simulink model "NOx_SCR_MIL_SIl_Model"  (R2019a)
settings: Solver=FixedStepDiscrete  StartTime=0.0  StopTime=500  FixedStep=0.1  RelTol=1e-3
undefined symbols (not defined in the file or in its folder): Actual_Injector_on, Flow_rate_min, Injector_off, injector_On_counter, Req_Downstrem_nox, Req_ON, Req_SCR_Bed_temp, Required_injector_On, Required_pressure, sigbuilder_block
settings Model: Creator=Kore  LastModifiedBy=Kore
settings ConfigComp: CovEnable=on  RecordCoverage=on  CovMetricSettings=dcmwe  CovModelRefEnable=on

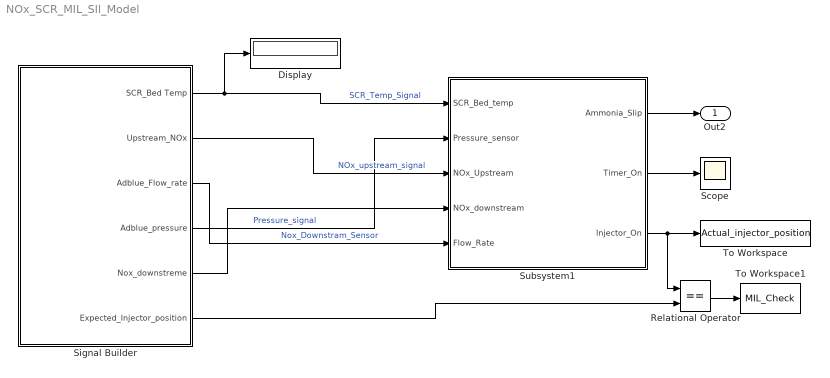
== system NOx_SCR_MIL_SIl_Model ==
  Display : Display
  Relational Operator : RelationalOperator  Operator===  OutDataTypeStr=boolean  RndMeth=Simplest
  Scope : Scope
  Signal Builder : Subsystem  Tag=STV Subsys  LoadFcn=sigbuilder_block('load');  StartFcn=sigbuilder_block('start');  StopFcn=sigbuilder_block('stop');  ClipboardFcn=sigbuilder_block('clipboard');  mask(Sigbuilder block){tuvar=[0:10]}
      mask help: Simulink:masks:SigbuilderBlock_MD
      mask init:
      | if ~strcmp(get_param(bdroot(gcbh),'SimulationStatus'),'stopped') tuvar = sigbuilder_block('maskInit'); end
      settings: CopyFcn=sigbuilder_block('copy');  DeleteFcn=sigbuilder_block('delete');  ModelCloseFcn=sigbuilder_block('modelClose');  PreSaveFcn=sigbuilder_block('preSave');  PauseFcn=sigbuilder_block('pause');  ContinueFcn=sigbuilder_block('continue');  NameChangeFcn=sigbuilder_block('namechange');  OpenFcn=sigbuilder_block('open',[437.6 153 550.4 359.25 ]);  CloseFcn=sigbuilder_block('close');
      mask Display: plot(0, 0, 100, 100,[2, 2, 32, 32, 2], [68, 8, 8, 68, 68],[32, 2], [38, 38], [32, 19, 2],[53, 60, 44], [32, 17, 17, 2],[16, 16, 31, 31]);txt = getActiveGroup(gcbh);text(2, 100, txt,'verticalAlignment', 'top');
  Subsystem1 : Subsystem
  To Workspace : ToWorkspace  VariableName=Actual_injector_position  SaveFormat=Timeseries  SampleTime=-1
  To Workspace1 : ToWorkspace  VariableName=MIL_Check  SaveFormat=Timeseries  SampleTime=-1
  Out2 : Outport
  wires:
  Subsystem1/3(Injector_On) -> Relational Operator/1, To Workspace/1
  Signal Builder/1(SCR_Bed Temp) -> Display/1, Subsystem1/1(SCR_Bed_temp)  "SCR_Temp_Signal"
  Subsystem1/1(Ammonia_Slip) -> Out2/1
  Signal Builder/2(Upstream_NOx) -> Subsystem1/3(NOx_Upstream)  "NOx_upstream_signal"
  Signal Builder/4(Adblue_pressure) -> Subsystem1/2(Pressure_sensor)  "Pressure_signal"
  Subsystem1/2(Timer_On) -> Scope/1
  Relational Operator/1 -> To Workspace1/1
  Signal Builder/6(Expected_Injector_position) -> Relational Operator/2
  Signal Builder/5(Nox_downstreme) -> Subsystem1/4(NOx_downstream)
  Signal Builder/3(Adblue_Flow_rate) -> Subsystem1/5(Flow_Rate)  "Nox_Downstram_Sensor"

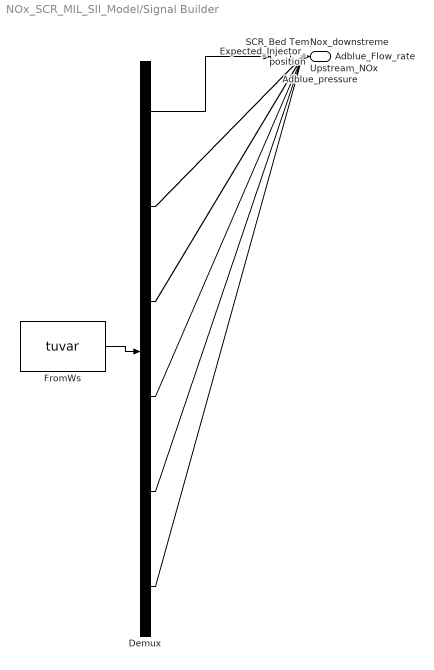
== system NOx_SCR_MIL_SIl_Model/Signal Builder ==
  Demux : Demux  Tag=STV Demux  Outputs=6
  FromWs : FromWorkspace  Tag=STV FromWs  VariableName=tuvar  SampleTime=0
      SigBuilderData=|
      | common.afterFinalStr = 'Extrapolate'
      | common.sampleTime = 0
      | dataSet.timeRange = [0 35.9]
      | dataSet.name = 'Sheet1'
      | sbobj.Name = 'Signal Builder'
      | sbobj.Groups.Name = 'Sheet1'
      | sbobj.Groups.Signals(1).Name = 'SCR_Bed Temp'
      | sbobj.Groups.Signals(1).XData = [0 0.1 0.2 0.3 0.4 0.5 0.6 0.7 0.8 0.9 1 1.1 1.2 1.3 1.4 1.5 1.6 1.7 1.8 1.9 2 2.1 2.2 2.3 2.4 2.5 2.6 2.7 2.8 2.9 3 3.1 3.2 3.3 3.4 3.5 3.6 3.7 3.8 3.9 4 4.1 4.2 4.3 4.4 4.5 4.6 4.7 4.8 4.9 5 5.1 5.2 5.3 5.4 5.5 5.6 5.7 5.8 5.9 6 6.1 6.2 6.3 6.4 6.5 6.6 6.7 6.8 6.9 7 7.1 7.2 7.3 7.4 7.5 7.6 7.7 7.8 7.9 8 8.1 8.2 8.3 8.4 8.5 8.6 8.7 8.8 8.9 9 9.1 9.2 9.3 9.4 9.5 9.6 9.7 9.8 9.9 10 10.1 10.2 10.3 10.4 10.5 10.6 10.7 10.8 10.9 11 11.1 11.2 11.3 11.4 11.5 11.6 11.7 11.8 11.9 12 12.1 12.2 12.3 12.4 12.5 12.6 12.7 12.8 12.9 13 13.1 13.2 13.3 13.4 13.5 13.6 13.7 13.8 13.9 14 14.1 14.2 14.3 14.4 14.5 14.6 14.7 14.8 14.9 15 15.1 15.2 15.3 15.4 15.5 15.6 15.7 15.8 15.9 16 16.1 16.2 16.3 16.4 16.5 16.6 16.7 16.8 16.9 17 17.1 17.2 17.3 17.4 17.5 17.6 17.7 17.8 17.9 18 18.1 18.2 18.3 18.4 18.5 18.6 18.7 18.8 18.9 19 19.1 19.2 19.3 19.4 19.5 19.6 19.7 19.8 19.9 20 20.1 20.2 20.3 20.4 20.5 20.6 20.7 20.8 20.9 21 21.1 21.2 21.3 21.4 21.5 21.6 21.7 21.8 21.9 22 22.1 22.2 22.3 22.4 22.5 22.6 22.7 22.8 22.9 23 23.1 23.2 23.3 23.4 23.5 23.6 23.7 23.8 23.9 24 24.1 24.2 24.3 24.4 24.5 24.6 24.7 24.8 24.9 25 25.1 25.2 25.3 25.4 25.5 25.6 25.7 25.8 25.9 26 26.1 26.2 26.3 26.4 26.5 26.6 26.7 26.8 26.9 27 27.1 27.2 27.3 27.4 27.5 27.6 27.7 27.8 27.9 28 28.1 28.2 28.3 28.4 28.5 28.6 28.7 28.8 28.9 29 29.1 29.2 29.3 29.4 29.5 29.6 29.7 29.8 29.9 30 30.1 30.2 30.3 30.4 30.5 30.6 30.7 30.8 30.9 31 31.1 31.2 31.3 31.4 31.5 31.6 31.7 31.8 31.9 32 32.1 32.2 32.3 32.4 32.5 32.6 32.7 32.8 32.9 33 33.1 33.2 33.3 33.4 33.5 33.6 33.7 33.8 33.9 34 34.1 34.2 34.3 34.4 34.5 34.6 34.7 34.8 34.9 35 35.1 35.2 35.3 35.4 35.5 35.6 35.7 35.8 35.9]
      | sbobj.Groups.Signals(1).YData = [1 10 20 30 40 50 60 70 80 90 100 110 120 130 140 150 160 170 180 190 200 210 220 230 240 250 260 270 280 290 300 310 320 330 340 350 360 370 380 390 400 410 420 430 440 450 460 470 480 490 500 510 520 530 540 550 560 570 580 590 600 610 620 630 640 650 660 670 10 20 30 40 50 60 70 80 90 100 110 120 130 140 150 160 170 180 190 200 210 220 230 240 250 260 270 280 290 300 310 320 330 340 350 360 370 380 390 400 410 420 430 440 450 460 470 480 490 500 510 520 530 540 550 560 570 580 590 600 610 620 630 640 650 660 670 10 20 30 40 50 60 70 80 90 100 110 120 130 140 150 160 170 180 190 200 210 220 230 240 250 260 270 280 290 300 310 320 330 340 350 360 370 380 390 400 410 420 430 440 450 460 470 480 490 500 510 520 530 540 550 560 570 580 590 600 610 620 630 640 650 660 670 10 20 30 40 50 60 70 80 90 100 110 120 130 140 150 160 170 180 190 200 210 220 230 240 250 260 270 280 290 300 310 320 330 340 350 360 370 380 390 400 410 420 430 440 450 460 470 480 490 500 510 520 530 540 550 560 570 580 590 600 610 620 630 640 650 660 670 200 205 210 215 220 225 230 235 240 245 250 255 260 265 270 275 280 285 290 295 300 305 310 315 320 325 330 335 340 345 350 355 360 365 370 375 380 385 390 395 400 405 410 415 420 425 430 435 440 445 450 455 460 465 470 475 480 485 490 495 500 505 510 515 520 525 530 535 540 545 550 555 560 565 570 575 580 585 590 595 600 605 610 615 620 625 630 635 640 645 650]
      | sbobj.Groups.Signals(2).Name = 'Upstream_NOx'
      | sbobj.Groups.Signals(2).XData = [0 0.1 0.2 0.3 0.4 0.5 0.6 0.7 0.8 0.9 1 1.1 1.2 1.3 1.4 1.5 1.6 1.7 1.8 1.9 2 2.1 2.2 2.3 2.4 2.5 2.6 2.7 2.8 2.9 3 3.1 3.2 3.3 3.4 3.5 3.6 3.7 3.8 3.9 4 4.1 4.2 4.3 4.4 4.5 4.6 4.7 4.8 4.9 5 5.1 5.2 5.3 5.4 5.5 5.6 5.7 5.8 5.9 6 6.1 6.2 6.3 6.4 6.5 6.6 6.7 6.8 6.9 7 7.1 7.2 7.3 7.4 7.5 7.6 7.7 7.8 7.9 8 8.1 8.2 8.3 8.4 8.5 8.6 8.7 8.8 8.9 9 9.1 9.2 9.3 9.4 9.5 9.6 9.7 9.8 9.9 10 10.1 10.2 10.3 10.4 10.5 10.6 10.7 10.8 10.9 11 11.1 11.2 11.3 11.4 11.5 11.6 11.7 11.8 11.9 12 12.1 12.2 12.3 12.4 12.5 12.6 12.7 12.8 12.9 13 13.1 13.2 13.3 13.4 13.5 13.6 13.7 13.8 13.9 14 14.1 14.2 14.3 14.4 14.5 14.6 14.7 14.8 14.9 15 15.1 15.2 15.3 15.4 15.5 15.6 15.7 15.8 15.9 16 16.1 16.2 16.3 16.4 16.5 16.6 16.7 16.8 16.9 17 17.1 17.2 17.3 17.4 17.5 17.6 17.7 17.8 17.9 18 18.1 18.2 18.3 18.4 18.5 18.6 18.7 18.8 18.9 19 19.1 19.2 19.3 19.4 19.5 19.6 19.7 19.8 19.9 20 20.1 20.2 20.3 20.4 20.5 20.6 20.7 20.8 20.9 21 21.1 21.2 21.3 21.4 21.5 21.6 21.7 21.8 21.9 22 22.1 22.2 22.3 22.4 22.5 22.6 22.7 22.8 22.9 23 23.1 23.2 23.3 23.4 23.5 23.6 23.7 23.8 23.9 24 24.1 24.2 24.3 24.4 24.5 24.6 24.7 24.8 24.9 25 25.1 25.2 25.3 25.4 25.5 25.6 25.7 25.8 25.9 26 26.1 26.2 26.3 26.4 26.5 26.6 26.7 26.8 26.9 27 27.1 27.2 27.3 27.4 27.5 27.6 27.7 27.8 27.9 28 28.1 28.2 28.3 28.4 28.5 28.6 28.7 28.8 28.9 29 29.1 29.2 29.3 29.4 29.5 29.6 29.7 29.8 29.9 30 30.1 30.2 30.3 30.4 30.5 30.6 30.7 30.8 30.9 31 31.1 31.2 31.3 31.4 31.5 31.6 31.7 31.8 31.9 32 32.1 32.2 32.3 32.4 32.5 32.6 32.7 32.8 32.9 33 33.1 33.2 33.3 33.4 33.5 33.6 33.7 33.8 33.9 34 34.1 34.2 34.3 34.4 34.5 34.6 34.7 34.8 34.9 35 35.1 35.2 35.3 35.4 35.5 35.6 35.7 35.8 35.9]
      | sbobj.Groups.Signals(2).YData = [10 70 77.6 80.4 86.4 99.6 108 117.6 127.2 136.8 149.3 158.3 ... (360 elements, 1x360)]
      | sbobj.Groups.Signals(3).Name = 'Adblue_Flow_rate'
      | sbobj.Groups.Signals(3).XData = [0 0.1 0.2 0.3 0.4 0.5 0.6 0.7 0.8 0.9 1 1.1 1.2 1.3 1.4 1.5 1.6 1.7 1.8 1.9 2 2.1 2.2 2.3 2.4 2.5 2.6 2.7 2.8 2.9 3 3.1 3.2 3.3 3.4 3.5 3.6 3.7 3.8 3.9 4 4.1 4.2 4.3 4.4 4.5 4.6 4.7 4.8 4.9 5 5.1 5.2 5.3 5.4 5.5 5.6 5.7 5.8 5.9 6 6.1 6.2 6.3 6.4 6.5 6.6 6.7 6.8 6.9 7 7.1 7.2 7.3 7.4 7.5 7.6 7.7 7.8 7.9 8 8.1 8.2 8.3 8.4 8.5 8.6 8.7 8.8 8.9 9 9.1 9.2 9.3 9.4 9.5 9.6 9.7 9.8 9.9 10 10.1 10.2 10.3 10.4 10.5 10.6 10.7 10.8 10.9 11 11.1 11.2 11.3 11.4 11.5 11.6 11.7 11.8 11.9 12 12.1 12.2 12.3 12.4 12.5 12.6 12.7 12.8 12.9 13 13.1 13.2 13.3 13.4 13.5 13.6 13.7 13.8 13.9 14 14.1 14.2 14.3 14.4 14.5 14.6 14.7 14.8 14.9 15 15.1 15.2 15.3 15.4 15.5 15.6 15.7 15.8 15.9 16 16.1 16.2 16.3 16.4 16.5 16.6 16.7 16.8 16.9 17 17.1 17.2 17.3 17.4 17.5 17.6 17.7 17.8 17.9 18 18.1 18.2 18.3 18.4 18.5 18.6 18.7 18.8 18.9 19 19.1 19.2 19.3 19.4 19.5 19.6 19.7 19.8 19.9 20 20.1 20.2 20.3 20.4 20.5 20.6 20.7 20.8 20.9 21 21.1 21.2 21.3 21.4 21.5 21.6 21.7 21.8 21.9 22 22.1 22.2 22.3 22.4 22.5 22.6 22.7 22.8 22.9 23 23.1 23.2 23.3 23.4 23.5 23.6 23.7 23.8 23.9 24 24.1 24.2 24.3 24.4 24.5 24.6 24.7 24.8 24.9 25 25.1 25.2 25.3 25.4 25.5 25.6 25.7 25.8 25.9 26 26.1 26.2 26.3 26.4 26.5 26.6 26.7 26.8 26.9 27 27.1 27.2 27.3 27.4 27.5 27.6 27.7 27.8 27.9 28 28.1 28.2 28.3 28.4 28.5 28.6 28.7 28.8 28.9 29 29.1 29.2 29.3 29.4 29.5 29.6 29.7 29.8 29.9 30 30.1 30.2 30.3 30.4 30.5 30.6 30.7 30.8 30.9 31 31.1 31.2 31.3 31.4 31.5 31.6 31.7 31.8 31.9 32 32.1 32.2 32.3 32.4 32.5 32.6 32.7 32.8 32.9 33 33.1 33.2 33.3 33.4 33.5 33.6 33.7 33.8 33.9 34 34.1 34.2 34.3 34.4 34.5 34.6 34.7 34.8 34.9 35 35.1 35.2 35.3 35.4 35.5 35.6 35.7 35.8 35.9]
      | sbobj.Groups.Signals(3).YData = [4 4 4 4 4 4 4 4 4 4.8 4.8 4.8 ... (360 elements, 1x360)]
      | sbobj.Groups.Signals(4).Name = 'Adblue_pressure'
      | sbobj.Groups.Signals(4).XData = [0 0.1 0.2 0.3 0.4 0.5 0.6 0.7 0.8 0.9 1 1.1 1.2 1.3 1.4 1.5 1.6 1.7 1.8 1.9 2 2.1 2.2 2.3 2.4 2.5 2.6 2.7 2.8 2.9 3 3.1 3.2 3.3 3.4 3.5 3.6 3.7 3.8 3.9 4 4.1 4.2 4.3 4.4 4.5 4.6 4.7 4.8 4.9 5 5.1 5.2 5.3 5.4 5.5 5.6 5.7 5.8 5.9 6 6.1 6.2 6.3 6.4 6.5 6.6 6.7 6.8 6.9 7 7.1 7.2 7.3 7.4 7.5 7.6 7.7 7.8 7.9 8 8.1 8.2 8.3 8.4 8.5 8.6 8.7 8.8 8.9 9 9.1 9.2 9.3 9.4 9.5 9.6 9.7 9.8 9.9 10 10.1 10.2 10.3 10.4 10.5 10.6 10.7 10.8 10.9 11 11.1 11.2 11.3 11.4 11.5 11.6 11.7 11.8 11.9 12 12.1 12.2 12.3 12.4 12.5 12.6 12.7 12.8 12.9 13 13.1 13.2 13.3 13.4 13.5 13.6 13.7 13.8 13.9 14 14.1 14.2 14.3 14.4 14.5 14.6 14.7 14.8 14.9 15 15.1 15.2 15.3 15.4 15.5 15.6 15.7 15.8 15.9 16 16.1 16.2 16.3 16.4 16.5 16.6 16.7 16.8 16.9 17 17.1 17.2 17.3 17.4 17.5 17.6 17.7 17.8 17.9 18 18.1 18.2 18.3 18.4 18.5 18.6 18.7 18.8 18.9 19 19.1 19.2 19.3 19.4 19.5 19.6 19.7 19.8 19.9 20 20.1 20.2 20.3 20.4 20.5 20.6 20.7 20.8 20.9 21 21.1 21.2 21.3 21.4 21.5 21.6 21.7 21.8 21.9 22 22.1 22.2 22.3 22.4 22.5 22.6 22.7 22.8 22.9 23 23.1 23.2 23.3 23.4 23.5 23.6 23.7 23.8 23.9 24 24.1 24.2 24.3 24.4 24.5 24.6 24.7 24.8 24.9 25 25.1 25.2 25.3 25.4 25.5 25.6 25.7 25.8 25.9 26 26.1 26.2 26.3 26.4 26.5 26.6 26.7 26.8 26.9 27 27.1 27.2 27.3 27.4 27.5 27.6 27.7 27.8 27.9 28 28.1 28.2 28.3 28.4 28.5 28.6 28.7 28.8 28.9 29 29.1 29.2 29.3 29.4 29.5 29.6 29.7 29.8 29.9 30 30.1 30.2 30.3 30.4 30.5 30.6 30.7 30.8 30.9 31 31.1 31.2 31.3 31.4 31.5 31.6 31.7 31.8 31.9 32 32.1 32.2 32.3 32.4 32.5 32.6 32.7 32.8 32.9 33 33.1 33.2 33.3 33.4 33.5 33.6 33.7 33.8 33.9 34 34.1 34.2 34.3 34.4 34.5 34.6 34.7 34.8 34.9 35 35.1 35.2 35.3 35.4 35.5 35.6 35.7 35.8 35.9]
      | sbobj.Groups.Signals(4).YData = [5.8 5.8 5.8 5.8 5.8 5.8 5.8 5.8 5.8 5.8 5.8 5.8 5.8 5.8 5.8 5.8 5.8 5.8 5.8 5.8 5.8 5.8 5.8 5.8 5.8 5.8 5.8 5.8 5.8 5.8 5.8 5.8 5.8 5.8 5.8 5.8 5.8 5.8 5.8 5.8 5.8 5.8 5.8 5.8 5.8 5.8 5.8 5.8 5.8 5.8 5.8 5.8 5.8 5.8 5.8 5.8 5.8 5.8 5.8 5.8 5.8 5.8 5.8 5.8 5.8 5.8 5.8 5.8 5.8 5.8 5.8 5.8 5.8 5.8 5.8 5.8 5.8 5.8 5.8 5.8 5.8 5.8 5.8 5.8 5.8 5.8 5.8 5.8 5.8 5.8 5.8 5.8 5.8 5.8 5.8 5.8 5.8 5.8 5.8 5.8 5.8 5.8 5.8 5.8 5.8 5.8 5.8 5.8 5.8 5.8 5.8 5.8 5.8 5.8 5.8 5.8 5.8 5.8 5.8 5.8 5.8 5.8 5.8 5.8 5.8 5.8 5.8 5.8 5.8 5.8 5.8 5.8 5.8 5.8 5.8 4.5 4.3 4.2 4.1 4.9 5 5.1 6 6.4 6.3 4.5 4.3 4.2 4.1 4.9 5 5.1 6 6.4 6.3 4.5 4.3 4.2 4.1 4.9 5 5.1 6 6.4 6.3 4.5 4.3 4.2 4.1 4.9 5 5.1 6 6.4 6.3 4.5 4.3 4.2 4.1 4.9 5 5.1 6 6.4 6.3 4.5 4.3 4.2 4.1 4.9 5 5.1 6 6.4 6.3 4.5 4.3 4.2 4.1 4.9 5 5.1 5.8 5.8 5.8 5.8 5.8 5.8 5.8 5.8 5.8 5.8 5.8 5.8 5.8 5.8 5.8 5.8 5.8 5.8 5.8 5.8 5.8 5.8 5.8 5.8 5.8 5.8 5.8 5.8 5.8 5.8 5.8 5.8 5.8 5.8 5.8 5.8 5.8 5.8 5.8 5.8 5.8 5.8 5.8 5.8 5.8 5.8 5.8 5.8 5.8 5.8 5.8 5.8 5.8 5.8 5.8 5.8 5.8 5.8 5.8 5.8 5.8 5.8 5.8 5.8 5.8 5.8 5.8 5.8 5.8 5.8 5.8 5.8 5.8 5.8 5.8 5.8 5.8 5.8 5.8 5.8 5.8 5.8 5.8 5.8 5.8 5.8 5.8 5.8 5.8 5.8 5.8 5.8 5.8 5.8 5.8 5.8 5.8 5.8 5.8 5.8 5.8 5.8 5.8 5.8 5.8 5.8 5.8 5.8 5.8 5.8 5.8 5.8 5.8 5.8 5.8 5.8 5.8 5.8 5.8 5.8 5.8 5.8 5.8 5.8 5.8 5.8 5.8 5.8 5.8 5.8 5.8 5.8 5.8 5.8 5.8 5.8 5.8 5.8 5.8 5.8 5.8 5.8 5.8 5.8 5.8 5.8 5.8 5.8 5.8 5.8 5.8 5.8 5.8 5.8 5.8 5.8 5.8 5.8]
      | sbobj.Groups.Signals(5).Name = 'Nox_downstreme'
      | sbobj.Groups.Signals(5).XData = [0 0.1 0.2 0.3 0.4 0.5 0.6 0.7 0.8 0.9 1 1.1 1.2 1.3 1.4 1.5 1.6 1.7 1.8 1.9 2 2.1 2.2 2.3 2.4 2.5 2.6 2.7 2.8 2.9 3 3.1 3.2 3.3 3.4 3.5 3.6 3.7 3.8 3.9 4 4.1 4.2 4.3 4.4 4.5 4.6 4.7 4.8 4.9 5 5.1 5.2 5.3 5.4 5.5 5.6 5.7 5.8 5.9 6 6.1 6.2 6.3 6.4 6.5 6.6 6.7 6.8 6.9 7 7.1 7.2 7.3 7.4 7.5 7.6 7.7 7.8 7.9 8 8.1 8.2 8.3 8.4 8.5 8.6 8.7 8.8 8.9 9 9.1 9.2 9.3 9.4 9.5 9.6 9.7 9.8 9.9 10 10.1 10.2 10.3 10.4 10.5 10.6 10.7 10.8 10.9 11 11.1 11.2 11.3 11.4 11.5 11.6 11.7 11.8 11.9 12 12.1 12.2 12.3 12.4 12.5 12.6 12.7 12.8 12.9 13 13.1 13.2 13.3 13.4 13.5 13.6 13.7 13.8 13.9 14 14.1 14.2 14.3 14.4 14.5 14.6 14.7 14.8 14.9 15 15.1 15.2 15.3 15.4 15.5 15.6 15.7 15.8 15.9 16 16.1 16.2 16.3 16.4 16.5 16.6 16.7 16.8 16.9 17 17.1 17.2 17.3 17.4 17.5 17.6 17.7 17.8 17.9 18 18.1 18.2 18.3 18.4 18.5 18.6 18.7 18.8 18.9 19 19.1 19.2 19.3 19.4 19.5 19.6 19.7 19.8 19.9 20 20.1 20.2 20.3 20.4 20.5 20.6 20.7 20.8 20.9 21 21.1 21.2 21.3 21.4 21.5 21.6 21.7 21.8 21.9 22 22.1 22.2 22.3 22.4 22.5 22.6 22.7 22.8 22.9 23 23.1 23.2 23.3 23.4 23.5 23.6 23.7 23.8 23.9 24 24.1 24.2 24.3 24.4 24.5 24.6 24.7 24.8 24.9 25 25.1 25.2 25.3 25.4 25.5 25.6 25.7 25.8 25.9 26 26.1 26.2 26.3 26.4 26.5 26.6 26.7 26.8 26.9 27 27.1 27.2 27.3 27.4 27.5 27.6 27.7 27.8 27.9 28 28.1 28.2 28.3 28.4 28.5 28.6 28.7 28.8 28.9 29 29.1 29.2 29.3 29.4 29.5 29.6 29.7 29.8 29.9 30 30.1 30.2 30.3 30.4 30.5 30.6 30.7 30.8 30.9 31 31.1 31.2 31.3 31.4 31.5 31.6 31.7 31.8 31.9 32 32.1 32.2 32.3 32.4 32.5 32.6 32.7 32.8 32.9 33 33.1 33.2 33.3 33.4 33.5 33.6 33.7 33.8 33.9 34 34.1 34.2 34.3 34.4 34.5 34.6 34.7 34.8 34.9 35 35.1 35.2 35.3 35.4 35.5 35.6 35.7 35.8 35.9]
      | sbobj.Groups.Signals(5).YData = [15 15 15 14 14 14 14 15 15 15 15 17 17 17 17 15 15 15 15 15 15 15 15 15 15 15 15 15 15 13 13 13 13 13 13 13 13 13 13 15 15 15 15 15 15 15 12 12 12 12 12 12 12 12 12 15 15 16 16 16 16 16 15 15 15 14 14 14 14 15 15 15 15 17 17 17 17 15 15 15 15 15 15 15 15 15 15 15 15 15 15 13 13 13 13 13 13 13 13 13 13 15 15 15 15 15 15 15 12 12 12 12 12 12 12 12 12 15 15 16 16 16 16 16 12 12 15 15 16 16 16 16 16 16 16 15 15 15 14 14 14 14 15 15 15 15 17 17 17 17 15 15 15 15 15 15 15 15 15 15 15 15 15 15 13 13 13 13 13 13 13 13 13 13 15 15 15 15 15 15 15 12 12 12 12 12 12 12 12 12 15 15 16 16 16 16 16 15 15 15 14 14 6 7 8 9 9 8 7 6 6 7 8 9 9 8 7 6 8 7 6 6 7 8 9 9 6 7 8 9 9 8 7 6 7 8 9 9 8 7 6 8 7 6 6 7 8 9 9 6 7 8 9 9 8 6 7 8 9 9 8 6 7 8 9 9 8 7 6 14 14 14 15 15 15 15 17 17 15 15 15 13 13 13 13 13 13 13 13 13 13 15 15 15 15 15 15 15 12 12 12 12 12 12 12 12 12 15 15 16 16 16 16 16 15 15 15 14 14 14 15 15 15 15 17 17 15 15 15 14 14 14 14 15 15 15 15 17 17 17 17 15 15 15 15 15 15 15 15 15 15 15 15 15 15 13 13 13 13 13]
      | sbobj.Groups.Signals(6).Name = 'Expected_Injector_position'
      | sbobj.Groups.Signals(6).XData = [0 0.1 0.2 0.3 0.4 0.5 0.6 0.7 0.8 0.9 1 1.1 1.2 1.3 1.4 1.5 1.6 1.7 1.8 1.9 2 2.1 2.2 2.3 2.4 2.5 2.6 2.7 2.8 2.9 3 3.1 3.2 3.3 3.4 3.5 3.6 3.7 3.8 3.9 4 4.1 4.2 4.3 4.4 4.5 4.6 4.7 4.8 4.9 5 5.1 5.2 5.3 5.4 5.5 5.6 5.7 5.8 5.9 6 6.1 6.2 6.3 6.4 6.5 6.6 6.7 6.8 6.9 7 7.1 7.2 7.3 7.4 7.5 7.6 7.7 7.8 7.9 8 8.1 8.2 8.3 8.4 8.5 8.6 8.7 8.8 8.9 9 9.1 9.2 9.3 9.4 9.5 9.6 9.7 9.8 9.9 10 10.1 10.2 10.3 10.4 10.5 10.6 10.7 10.8 10.9 11 11.1 11.2 11.3 11.4 11.5 11.6 11.7 11.8 11.9 12 12.1 12.2 12.3 12.4 12.5 12.6 12.7 12.8 12.9 13 13.1 13.2 13.3 13.4 13.5 13.6 13.7 13.8 13.9 14 14.1 14.2 14.3 14.4 14.5 14.6 14.7 14.8 14.9 15 15.1 15.2 15.3 15.4 15.5 15.6 15.7 15.8 15.9 16 16.1 16.2 16.3 16.4 16.5 16.6 16.7 16.8 16.9 17 17.1 17.2 17.3 17.4 17.5 17.6 17.7 17.8 17.9 18 18.1 18.2 18.3 18.4 18.5 18.6 18.7 18.8 18.9 19 19.1 19.2 19.3 19.4 19.5 19.6 19.7 19.8 19.9 20 20.1 20.2 20.3 20.4 20.5 20.6 20.7 20.8 20.9 21 21.1 21.2 21.3 21.4 21.5 21.6 21.7 21.8 21.9 22 22.1 22.2 22.3 22.4 22.5 22.6 22.7 22.8 22.9 23 23.1 23.2 23.3 23.4 23.5 23.6 23.7 23.8 23.9 24 24.1 24.2 24.3 24.4 24.5 24.6 24.7 24.8 24.9 25 25.1 25.2 25.3 25.4 25.5 25.6 25.7 25.8 25.9 26 26.1 26.2 26.3 26.4 26.5 26.6 26.7 26.8 26.9 27 27.1 27.2 27.3 27.4 27.5 27.6 27.7 27.8 27.9 28 28.1 28.2 28.3 28.4 28.5 28.6 28.7 28.8 28.9 29 29.1 29.2 29.3 29.4 29.5 29.6 29.7 29.8 29.9 30 30.1 30.2 30.3 30.4 30.5 30.6 30.7 30.8 30.9 31 31.1 31.2 31.3 31.4 31.5 31.6 31.7 31.8 31.9 32 32.1 32.2 32.3 32.4 32.5 32.6 32.7 32.8 32.9 33 33.1 33.2 33.3 33.4 33.5 33.6 33.7 33.8 33.9 34 34.1 34.2 34.3 34.4 34.5 34.6 34.7 34.8 34.9 35 35.1 35.2 35.3 35.4 35.5 35.6 35.7 35.8 35.9]
      | sbobj.Groups.Signals(6).YData = [0 0 0 0 0 0 0 0 0 0 0 0 0 0 0 0 0 0 0 0 1 1 1 1 1 1 1 1 1 1 1 1 1 1 1 1 1 1 1 1 1 1 1 1 1 1 1 1 1 1 1 1 1 1 1 1 1 1 1 1 1 1 1 1 1 1 1 1 0 0 0 0 0 0 0 0 0 0 0 0 0 0 0 0 0 0 0 0 0 0 0 0 0 0 0 0 0 0 0 0 0 0 0 0 0 0 0 0 0 0 0 0 0 0 0 0 0 0 0 0 0 0 0 0 0 0 0 0 0 0 0 0 0 0 0 0 0 0 0 0 0 0 0 0 0 0 0 0 0 0 0 0 0 0 0 0 0 0 0 0 0 0 0 0 0 0 0 0 0 0 0 0 0 0 0 0 0 0 0 0 0 0 0 0 0 0 0 0 0 0 0 0 0 0 0 0 0 0 0 0 0 0 0 0 0 0 0 0 0 0 0 0 0 0 0 0 0 0 0 0 0 0 0 0 0 0 0 0 0 0 0 0 0 0 0 0 0 0 0 0 0 0 0 0 0 0 0 0 0 0 0 0 0 0 0 0 0 0 0 0 0 0 0 0 0 0 0 0 0 1 1 1 1 1 1 1 1 1 1 1 1 1 1 1 1 1 1 1 1 1 1 1 1 1 1 1 1 1 1 1 1 1 1 1 1 1 1 1 1 1 1 1 1 1 1 1 1 1 1 1 1 1 1 1 1 1 1 1 1 1 1 1 1 1 1 1 1 1 1 1 1 1 1 1 1 1 1 1 1 1 1 1 1 1 1 1 1 1 1 1]
      | sbobj.Groups.TimeRange = [0 35.9]
  SCR_Bed Temp : Outport  Tag=STV Outport
  Upstream_NOx : Outport  Tag=STV Outport  Port=2
  Adblue_Flow_rate : Outport  Tag=STV Outport  Port=3
  Adblue_pressure : Outport  Tag=STV Outport  Port=4
  Nox_downstreme : Outport  Tag=STV Outport  Port=5
  Expected_Injector_position : Outport  Tag=STV Outport  Port=6
  wires:
  Demux/1 -> SCR_Bed Temp/1
  FromWs/1 -> Demux/1
  Demux/2 -> Upstream_NOx/1
  Demux/3 -> Adblue_Flow_rate/1
  Demux/4 -> Adblue_pressure/1
  Demux/5 -> Nox_downstreme/1
  Demux/6 -> Expected_Injector_position/1

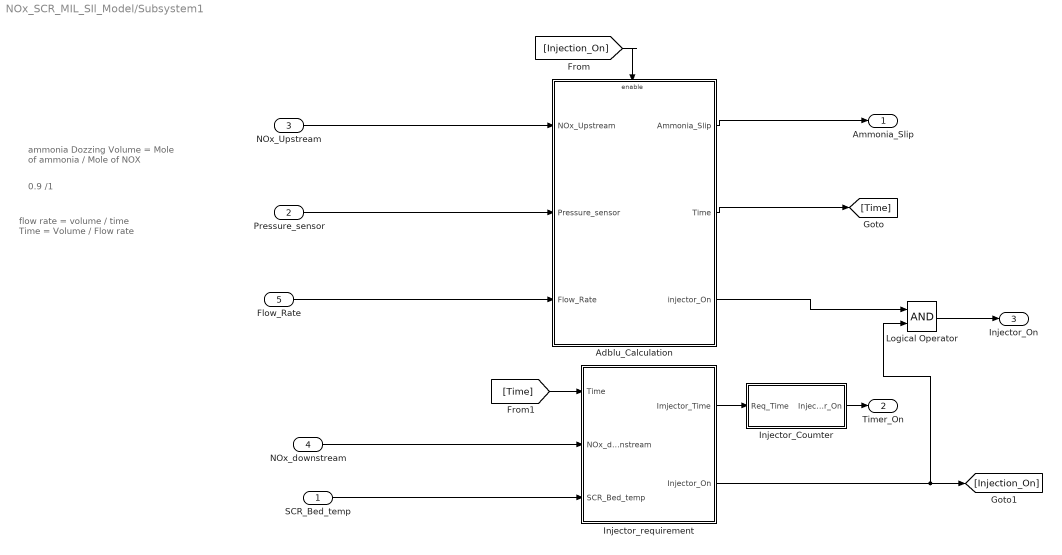
== system NOx_SCR_MIL_SIl_Model/Subsystem1 ==
  note: 0.9 /1
  note: ammonia Dozzing Volume =
      |  Mole of ammonia / Mole of NOX
  note: flow rate = volume / time
      |
      | Time = Volume / Flow rate
  SCR_Bed_temp : Inport
  Pressure_sensor : Inport  Port=2
  NOx_Upstream : Inport  Port=3
  NOx_downstream : Inport  Port=4
  Flow_Rate : Inport  Port=5
  Adblu_Calculation : Subsystem
  Injector_Coumter : Subsystem
  Injector_requirement : Subsystem
  Logical Operator : Logic  AllPortsSameDT=off  OutDataTypeStr=boolean
  Ammonia_Slip : Outport
  Timer_On : Outport  Port=2
  Injector_On : Outport  Port=3
  wires:
  NOx_Upstream/1 -> Adblu_Calculation/1(NOx_Upstream)
  Pressure_sensor/1 -> Adblu_Calculation/2(Pressure_sensor)
  Adblu_Calculation/1(Ammonia_Slip) -> Ammonia_Slip/1
  NOx_downstream/1 -> Injector_requirement/2(NOx_downstream)
  [Injection_On] -> Adblu_Calculation/Enable
  Injector_Coumter/1(Injector_On) -> Timer_On/1
  SCR_Bed_temp/1 -> Injector_requirement/3(SCR_Bed_temp)
  Injector_requirement/1(Imjector_Time) -> Injector_Coumter/1(Req_Time)
  Adblu_Calculation/2(Time) -> [Time]
  [Time] -> Injector_requirement/1(Time)
  Injector_requirement/2(Injector_On) -> Logical Operator/2, [Injection_On]
  Flow_Rate/1 -> Adblu_Calculation/3(Flow_Rate)
  Adblu_Calculation/3(injector_On) -> Logical Operator/1
  Logical Operator/1 -> Injector_On/1

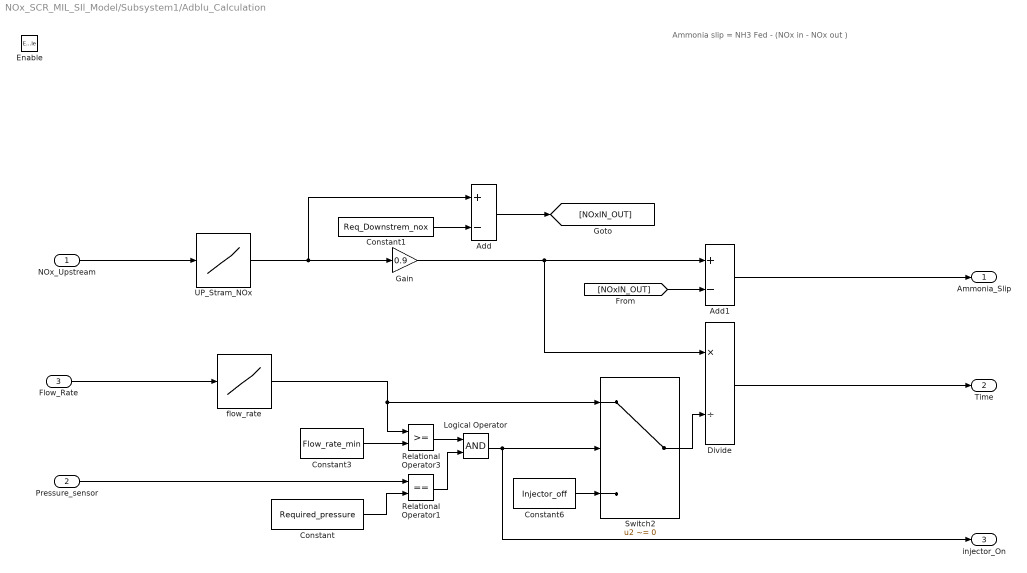
== system NOx_SCR_MIL_SIl_Model/Subsystem1/Adblu_Calculation ==
  note: Ammonia slip = NH3 Fed - (NOx in - NOx out )
  NOx_Upstream : Inport
  Pressure_sensor : Inport  Port=2
  Flow_Rate : Inport  Port=3
  Enable : EnablePort  StatesWhenEnabling=reset
  Add : Sum  Inputs=+-
  Add1 : Sum  Inputs=+-
  Constant : Constant  Value=Required_pressure
  Constant1 : Constant  Value=Req_Downstrem_nox
  Constant3 : Constant  Value=Flow_rate_min
  Constant6 : Constant  Value=Injector_off
  Divide : Product  Inputs=*/  OutDataTypeStr=double  RndMeth=Round
  Gain : Gain  Gain=0.9
  Logical Operator : Logic  AllPortsSameDT=off  OutDataTypeStr=boolean
  Relational Operator1 : RelationalOperator  Operator===  OutDataTypeStr=boolean  RndMeth=Simplest
  Relational Operator3 : RelationalOperator  OutDataTypeStr=boolean  RndMeth=Simplest
  Switch2 : Switch  Criteria=u2 ~= 0
  UP_Stram_NOx : Lookup_n-D  NumberOfTableDimensions=1  BreakpointsForDimension1=[1:5:650]  BreakpointsForDimension2=[1:1:500]  BreakpointsForDimension1DataTypeStr=double  Table=[1:5:650]  TableDataTypeStr=double  IntermediateResultsDataTypeStr=double  InternalRulePriority=Speed  OutDataTypeStr=double  RndMeth=Simplest  FractionDataTypeStr=double  InputSameDT=on
  flow_rate : Lookup_n-D  NumberOfTableDimensions=1  BreakpointsForDimension1=|  BreakpointsForDimension2=[1:1:500]  BreakpointsForDimension1DataTypeStr=double  Table=|  TableDataTypeStr=double  IntermediateResultsDataTypeStr=double  InternalRulePriority=Speed  OutDataTypeStr=double  RndMeth=Simplest  FractionDataTypeStr=double  InputSameDT=on
      BreakpointsForDimension1=|
      | [10
      | 70
      | 77.6
      | 80.4
      | 86.4
      | 99.6
      | 108
      | 117.6
      | 127.2
      | 136.8
      | 149.3
      | 158.3
      | 163.3
      | 168.3
      | 175.3
      | 181.5
      | 187.7
      | 193.9
      | 200.1
      | 206.3
      | 212.85
      | 223.5
      | 233.15
      | 242.8
      | 255.45
      | 264.9
      | 275.35
      | 285.8
      | 296.25
      | 306.7
      | 317.15
      | 327.6
      | 338.05
      | 348.5
      | 358.95
      | 369.4
      | 379.85
      | 390.3
      | 400.75
      | 411.2
      | 421.65
      | 432.1
      | 442.55
      | 453
      | 463.45
      | 473.9
      | 484.35
      | 494.8
      | 505.25
      | 515.7
      | 526.15
      | 536.6
      | 547.05
      | 557.5
      | 567.95
      | 578.4
      | 588.85
      | 599.3
      | 609.75
      | 620.2
      | 630.65
      | 641.1
      | 651.55
      | 662
      | 672.45
      | 682.9
      | 693.35
      | 703.8
      | ]
      Table=|
      | [3
      | 3
      | 3
      | 3
      | 3
      | 4
      | 4
      | 4
      | 4
      | 4.8
      | 4.8
      | 4.8
      | 4.8
      | 4.8
      | 4.8
      | 4.8
      | 4.8
      | 4.8
      | 4.8
      | 4.8
      | 4.8
      | 5.8
      | 6.4
      | 7.3
      | 8.1
      | 8.9
      | 9.7
      | 10.5
      | 11.3
      | 12.1
      | 12.9
      | 13.7
      | 14.5
      | 15.3
      | 16.1
      | 16.9
      | 17.7
      | 18.5
      | 19.3
      | 20.1
      | 20.9
      | 21.7
      | 22.5
      | 23.3
      | 24.1
      | 24.9
      | 25.7
      | 26.5
      | 27.3
      | 27.3
      | 27.3
      | 28.1
      | 28.1
      | 28.1
      | 28.1
      | 28.9
      | 28.9
      | 28.9
      | 28.9
      | 28.9
      | 28.9
      | 29.7
      | 29.7
      | 29.7
      | 29.7
      | 30.0
      | 30.0
      | 30.0]
  Ammonia_Slip : Outport
  Time : Outport  Port=2
  injector_On : Outport  Port=3
  wires:
  Pressure_sensor/1 -> Relational Operator1/1
  Add/1 -> [NOxIN_OUT]
  Constant1/1 -> Add/2
  Relational Operator1/1 -> Logical Operator/2
  Constant/1 -> Relational Operator1/2
  UP_Stram_NOx/1 -> Gain/1, Add/1
  Constant3/1 -> Relational Operator3/2
  Relational Operator3/1 -> Logical Operator/1
  Constant6/1 -> Switch2/3
  Switch2/1 -> Divide/2
  Logical Operator/1 -> injector_On/1, Switch2/2
  [NOxIN_OUT] -> Add1/2
  flow_rate/1 -> Relational Operator3/1, Switch2/1
  NOx_Upstream/1 -> UP_Stram_NOx/1
  Add1/1 -> Ammonia_Slip/1
  Gain/1 -> Divide/1, Add1/1
  Divide/1 -> Time/1
  Flow_Rate/1 -> flow_rate/1

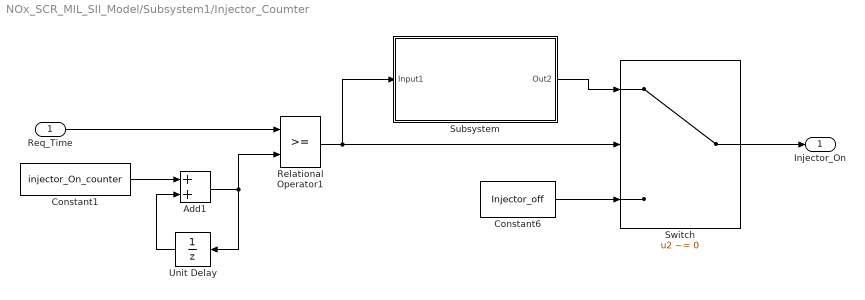
== system NOx_SCR_MIL_SIl_Model/Subsystem1/Injector_Coumter ==
  Req_Time : Inport
  Add1 : Sum
  Constant1 : Constant  Value=injector_On_counter
  Constant6 : Constant  Value=Injector_off
  Relational Operator1 : RelationalOperator  OutDataTypeStr=boolean  RndMeth=Simplest
  Subsystem : Subsystem
  Switch : Switch  Criteria=u2 ~= 0
  Unit Delay : UnitDelay  SampleTime=-1  HasFrameUpgradeWarning=on
  Injector_On : Outport
  wires:
  Constant6/1 -> Switch/3
  Unit Delay/1 -> Add1/2
  Constant1/1 -> Add1/1
  Add1/1 -> Unit Delay/1, Relational Operator1/2
  Subsystem/1(Out2) -> Switch/1
  Req_Time/1 -> Relational Operator1/1
  Switch/1 -> Injector_On/1
  Relational Operator1/1 -> Subsystem/1(Input1), Switch/2

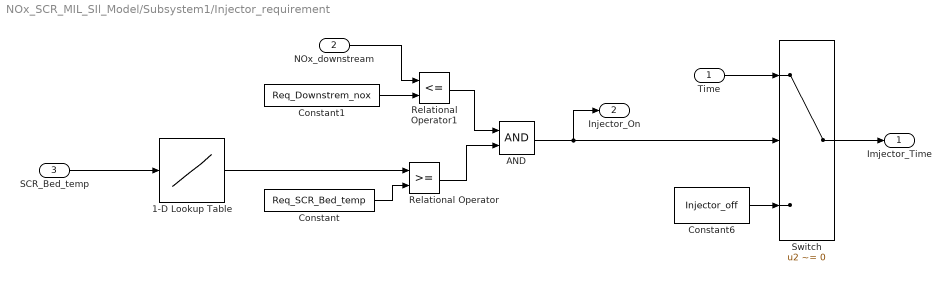
== system NOx_SCR_MIL_SIl_Model/Subsystem1/Injector_requirement ==
  Time : Inport
  NOx_downstream : Inport  Port=2
  SCR_Bed_temp : Inport  Port=3
  1-D Lookup Table : Lookup_n-D  NumberOfTableDimensions=1  BreakpointsForDimension1=[1:10:650]  BreakpointsForDimension2=[1:1:500]  BreakpointsForDimension1DataTypeStr=double  Table=[1:10:650]  TableDataTypeStr=double  IntermediateResultsDataTypeStr=double  InternalRulePriority=Speed  OutDataTypeStr=double  RndMeth=Simplest  FractionDataTypeStr=double  InputSameDT=on
  AND : Logic  AllPortsSameDT=off  OutDataTypeStr=boolean
  Constant : Constant  Value=Req_SCR_Bed_temp
  Constant1 : Constant  Value=Req_Downstrem_nox
  Constant6 : Constant  Value=Injector_off
  Relational Operator : RelationalOperator  OutDataTypeStr=boolean  RndMeth=Simplest
  Relational Operator1 : RelationalOperator  Operator=<=  OutDataTypeStr=boolean  RndMeth=Simplest
  Switch : Switch  Criteria=u2 ~= 0
  Imjector_Time : Outport
  Injector_On : Outport  Port=2
  wires:
  Constant1/1 -> Relational Operator1/2
  Constant/1 -> Relational Operator/2
  Constant6/1 -> Switch/3
  1-D Lookup Table/1 -> Relational Operator/1
  AND/1 -> Injector_On/1, Switch/2
  Time/1 -> Switch/1
  Relational Operator1/1 -> AND/1
  Relational Operator/1 -> AND/2
  SCR_Bed_temp/1 -> 1-D Lookup Table/1
  Switch/1 -> Imjector_Time/1
  NOx_downstream/1 -> Relational Operator1/1

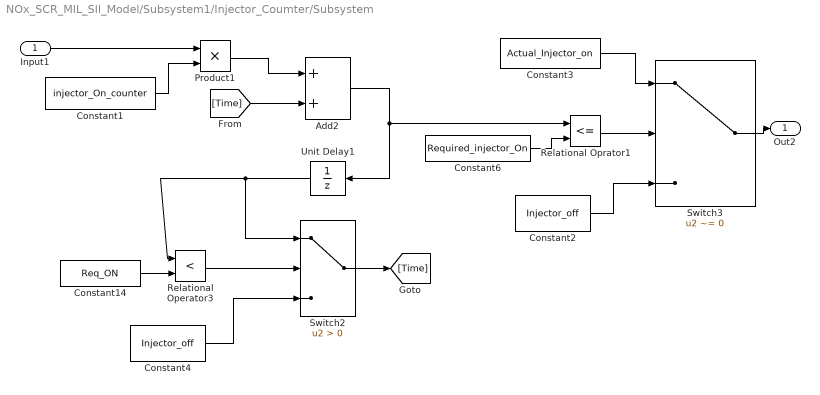
== system NOx_SCR_MIL_SIl_Model/Subsystem1/Injector_Coumter/Subsystem ==
  Input1 : Inport
  Add2 : Sum
  Constant1 : Constant  Value=injector_On_counter
  Constant14 : Constant  Value=Req_ON
  Constant2 : Constant  Value=Injector_off
  Constant3 : Constant  Value=Actual_Injector_on
  Constant4 : Constant  Value=Injector_off
  Constant6 : Constant  Value=Required_injector_On
  Product1 : Product
  Relational Operator3 : RelationalOperator  Operator=<  OutDataTypeStr=boolean  RndMeth=Simplest
  Relational Oprator1 : RelationalOperator  Operator=<=  OutDataTypeStr=boolean  RndMeth=Simplest
  Switch2 : Switch  Criteria=u2 > Threshold
  Switch3 : Switch  Criteria=u2 ~= 0
  Unit Delay1 : UnitDelay  SampleTime=-1  HasFrameUpgradeWarning=on
  Out2 : Outport
  wires:
  Unit Delay1/1 -> Relational Operator3/1, Switch2/1
  Relational Operator3/1 -> Switch2/2
  Constant3/1 -> Switch3/1
  Switch3/1 -> Out2/1
  Constant6/1 -> Relational Oprator1/2
  Constant1/1 -> Product1/2
  Switch2/1 -> [Time]
  Product1/1 -> Add2/1
  Constant14/1 -> Relational Operator3/2
  Constant4/1 -> Switch2/3
  Input1/1 -> Product1/1
  Constant2/1 -> Switch3/3
  [Time] -> Add2/2
  Relational Oprator1/1 -> Switch3/2
  Add2/1 -> Relational Oprator1/1, Unit Delay1/1
